simulink model "ButtonHold2SecondsCheck_v2"  (R2025a)
settings: Solver=FixedStepDiscrete  StartTime=0.0  StopTime=10.0  FixedStep=0.02  RelTol=1e-3
libraries: simulink x1
settings Model: Creator=mahij  LastModifiedBy=mahij

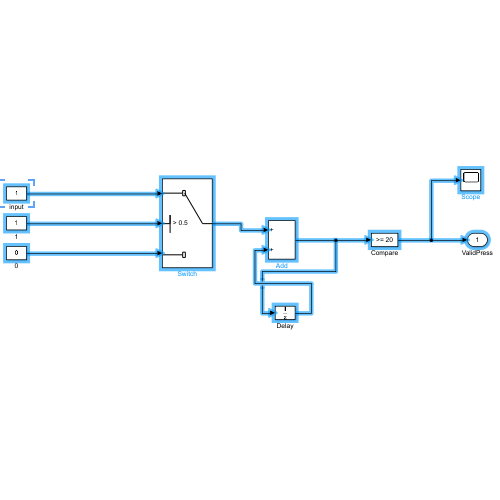
[thumbnail: Simulink's stored preview of the top-level diagram]
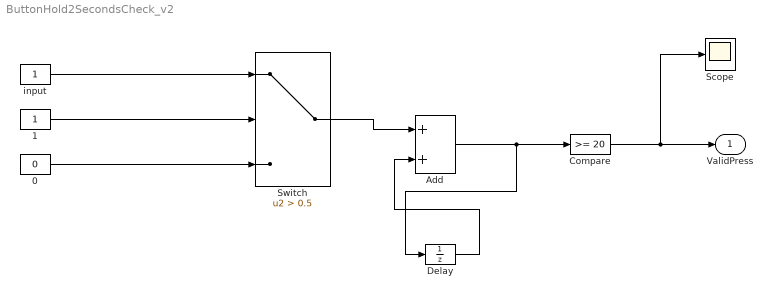
== system ButtonHold2SecondsCheck_v2 ==
  0 : Constant  Value=0
  1 : Constant
  Add : Sum
  Compare : simulink/Logic and Bit Operations/Compare To Constant  relop=>=  const=20  OutDataTypeStr=boolean
  Delay : UnitDelay  SampleTime=0.1  HasFrameUpgradeWarning=on
  Scope : Scope
      settings: ActiveDisplayYMinimum=-0.12499999999999997  ActiveDisplayYMaximum=1.125
  Switch : Switch  Criteria=u2 > Threshold  Threshold=0.5  SaturateOnIntegerOverflow=off  InputSameDT=off
  input : Constant
  ValidPress : Outport
  wires:
  input/1 -> Switch/1
  1/1 -> Switch/2
  0/1 -> Switch/3
  Switch/1 -> Add/1
  Delay/1 -> Add/2
  Add/1 -> Compare/1, Delay/1
  Compare/1 -> Scope/1, ValidPress/1
